simulink model "modPowerSys"  (R2019b)
settings: Solver=ode15s  StartTime=StartTime  StopTime=StopTime  FixedStep=FixedStepSize  MaxStep=0.01  RelTol=1e-3  EnableMultiTasking=on
values from neighbouring files (symbols this model uses):
  D = 0.5 * D    [main.m]
  dP = Pset(3)/Pbase    [main.m]
  Ki = 2    [main.m]
  KOnline = sum(kset.*Punit)/Pbase    [main.m]
  Kp = 20    [main.m]
  M = 0.5 * M    [main.m]
  R = 0.05    [main.m]
  TCH = 2    [main.m]
settings Model: ExtModeAutoUpdateStatusClock=off  Creator=posq  LastModifiedBy=edxu96
settings DataIOCC: LimitDataPoints=on  SaveFormat=Array  SignalLoggingSaveFormat=ModelDataLogs  SaveTime=off  ReturnWorkspaceOutputs=off
settings OptimizationCC: InitFltsAndDblsToZero=on  LifeSpan=inf
settings DebuggingCC: SaveWithParameterizedLinksMsg=none  UnderspecifiedInitializationDetection=Classic  MergeDetectMultiDrivingBlocksExec=none  SolverPrmCheckMsg=warning  MultiTaskCondExecSysMsg=none  FcnCallInpInsideContextMsg=warning  StateNameClashWarn=warning  SFUnexpectedBacktrackingDiag=warning  SFNoUnconditionalDefaultTransitionDiag=warning  SFExecutionAtInitializationDiag=none  ArithmeticOperatorsInVariantConditions=warning
settings HardwareCC: ProdBitPerPointer=32  ProdBitPerSizeT=32  ProdBitPerPtrDiffT=32  ProdLargestAtomicFloat=None  ProdIntDivRoundTo=Undefined  ProdEndianess=Unspecified  ProdWordSize=32  ProdHWDeviceType=32-bit Generic
settings ModelReferenceCC: PropagateSignalLabelsOutOfModel=off
settings SFSimCC: SimUseLocalCustomCode=off  CustomCodeUndefinedFunction=UseInterfaceOnly
settings RTWCC: RTWUseLocalCustomCode=off
settings CodeAppCC: StateflowObjectComments=on
settings GRTTargetCC: TargetLangStandard=C89/C90 (ANSI)  GeneratePreprocessorConditionals=Disable all  CombineOutputUpdateFcns=off  GRTInterface=on
settings ConfigComp: CovMetricSettings=dw  CovHtmlReporting=on  CovSaveCumulativeToWorkspaceVar=on  CovSaveSingleToWorkspaceVar=on  CovExternalEMLEnable=off

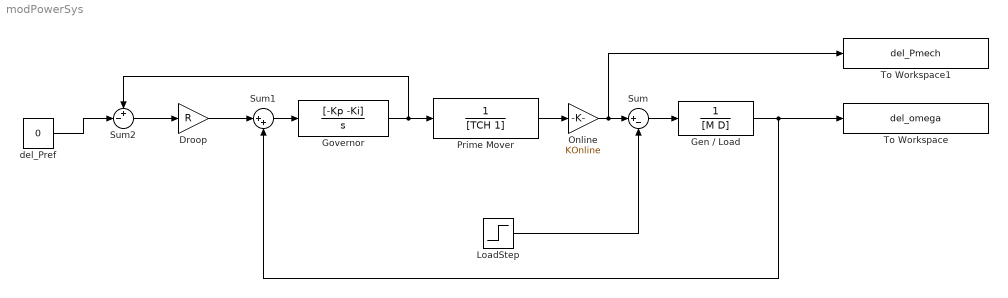
== system modPowerSys ==
  Droop : Gain  Gain=R
  Gen / Load : TransferFcn  Denominator=[M D]
  Governor : TransferFcn  Numerator=[-Kp -Ki]  Denominator=[1 0]
  LoadStep : Step  Time=0  After=dP  SampleTime=0
  Online : Gain  Gain=KOnline
  Prime Mover : TransferFcn  Denominator=[TCH 1]
  Sum : Sum  Inputs=|+-
  Sum1 : Sum  Inputs=|++
  Sum2 : Sum  Inputs=+-|
  To Workspace : ToWorkspace  VariableName=del_omega  SaveFormat=Structure With Time  SampleTime=-1
  To Workspace1 : ToWorkspace  VariableName=del_Pmech  SaveFormat=Structure With Time  SampleTime=-1
  del_Pref : Constant  Value=0
  wires:
  Gen / Load/1 -> To Workspace/1, Sum1/2
  Sum/1 -> Gen / Load/1
  LoadStep/1 -> Sum/2
  Governor/1 -> Sum2/1, Prime Mover/1
  Sum1/1 -> Governor/1
  Droop/1 -> Sum1/1
  Prime Mover/1 -> Online/1
  Online/1 -> To Workspace1/1, Sum/1
  del_Pref/1 -> Sum2/2
  Sum2/1 -> Droop/1
